simulink model "experiment_simulation"  (R2023b)
settings: Solver=VariableStepAuto  StartTime=0.0  StopTime=27  RelTol=1e-3
InitFcn:
  | parameters
model workspace (MAT data in the model file):
  trajectory_a = [-1.52409846931  1.70613035573  0.374243089925  1.5344612197  -0.302096275649  0.429029543536  -1.71694567009  1.69908972473  0.568317664567  -1.58200132841; 0.800900294758  -0.416782684687  -1.66038099689  -1.1420845298  -1.00480440985  -1.09338745015  0.812017564072  1.01661034087  0.189146535455  0.213933679737; 0.522291166812  1.94182780206  0.53711281193  0.401822450123  1.63674782832  0.283346535529  -0.658320315012  1.82855663324  -0.240307510879  0.406170374063; 0.881049446282  0.715113366686  -1.14896395959  -1.67350649982  -0.902082368458  1.47007354587  0.23742826959  -0.141488915891  -0.278796396878  1.09594368008; 0.615681685123  0.630917086666  -1.35591638166  -0.270492692225  0.0203443374221  -0.49867087628  -0.0785110876565  -0.630314388932  1.10858576056  -0.464224550441; 0.846225707965  -0.0762663704322  0.916720888486  1.75023695585  0.0690176102037  1.61227499451  -1.12722943148  1.49287736069  -1.66922827228  -0.138386333717; -1.91228070877  1.23312220014  -1.28316199684  -1.33843101258  -1.27358613135  0.765746253245  -1.14494592309  -0.807580560907  1.07334058824  0.00460037858408]
  trajectory_b = [1.63785922603  -1.76858838765  -0.252992287028  0.289018982285  0.260268639109  1.29526626891  -1.49560469007  -0.799532889865  -1.99151190067  1.80442943156; 1.06519745333  1.00521664875  -1.44454065144  -0.602721829429  -1.39463775801  -0.0131172869683  1.23460901165  0.531475173765  0.753605990771  0.558280871421; 0.917286904974  1.43938283234  0.507821517658  -1.27763450836  0.29322618533  -1.34573537446  1.6242069423  -1.69062885947  -0.645861399433  0.322470189589; -0.0990593700309  1.2212819449  0.123112563899  -1.09075867343  0.837939900786  -1.40546978718  0.632464724894  0.53593019156  -1.08277499414  -1.27108793891; -1.33458996905  -1.40157163353  -1.18901040903  1.81983560726  -1.93636664476  1.83005740068  -1.89723085852  1.88444265238  -0.809617292966  0.100292316878; 1.44935684592  1.58561961386  -1.24395777836  0.642878229792  1.76492375149  1.90282850268  -1.56825898793  -1.28440308791  0.986205708528  -1.80212590987; -1.71486047215  -0.0434979217147  1.39957528496  1.98816577551  -1.98242954967  0.170429856236  1.44539270567  1.63655609788  1.38140224911  1.51549153855]
values from neighbouring files (symbols this model uses):
  m = length(U)-1    [bspline_findspan.m]
  param_robot = load_mu(param_robot, mu)    [parameters.m]
undefined symbols (not defined in the file or in its folder): par, param_initial_condition, param_sensor, X, Y, Z
libraries: nesl_utility x308, sm_lib x269, simulink_extras x1
(part 1 of 4)
settings Model: Creator=cha  LastModifiedBy=simon
settings SolverCC: AlgebraicLoopSolver=TrustRegion
settings DataIOCC: ReturnWorkspaceOutputs=off
settings DebuggingCC: UnconnectedLineMsg=warning  ArithmeticOperatorsInVariantConditions=warning
settings ModelReferenceCC: EnableRefExpFcnMdlSchedulingChecks=on
settings SFSimCC: SimUseLocalCustomCode=off  CustomCodeUndefinedFunction=UseInterfaceOnly
settings RTWCC: RTWUseLocalCustomCode=off
settings ExplorerConfigSet: InternalSimMechanicsExplorerSettings="<ExplorerConfiguration><canonicalview>default</canonicalview><AnimationSetting><BasePlaybackSpeed>1.0</BasePlaybackSpeed><PlaybackSpeedFactor>1.0</PlaybackSpeedFactor></AnimationSetting><TilePanel><TileInfo><Tiles Columns=\"1\" Count=\"1\" Rows=\"1\"><Column Weight=\"1\"/><Row Weight=\"1\"/><Tile Height=\"1\" Width=\"1\" X=\"0\" Y=\"0\"/></Tiles></TileInfo><SceneInfo><SceneViewer><BGColor><R>0.60000002384185791</R><G>0.60000002384185791</G><B>0.60000002384185791</B></BGColor><Camera><DoPerspective>off</DoPerspective><Position><X>0.880405044047670393</X><Y>-0.700942246579231321</Y><Z>1.1419415318535151</Z></Position><Center><X>0.329533173940033675</X><Y>0.0559357238790175043</Y><Z>0.725925616444012989</Z></Center><Up><X>-0.2202813222044534</X><Y>0.341822804085735843</Y><Z>0.913582678083830313</Z></Up><ViewLimDist>1</ViewLimDist><YLim>0.787222366901565107</YLim><XLim>1.5531684536166015</XLim></Camera></SceneViewer></SceneInfo></TilePanel><MechEditorPanel><Cameras/><GfxPanelCameraMap/><VideoCreator><PlaybackSpeedRatio>1.0</PlaybackSpeedRatio><FrameRate>30</FrameRate><VideoFormat>Motion JPEG AVI</VideoFormat><FrameSize>auto</FrameSize></VideoCreator></MechEditorPanel></ExplorerConfiguration>"

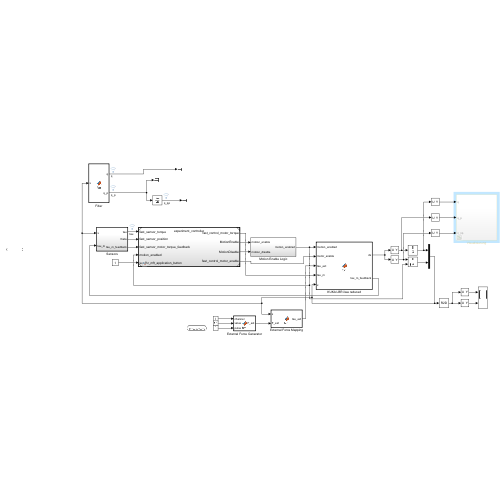
[thumbnail: Simulink's stored preview of the top-level diagram]
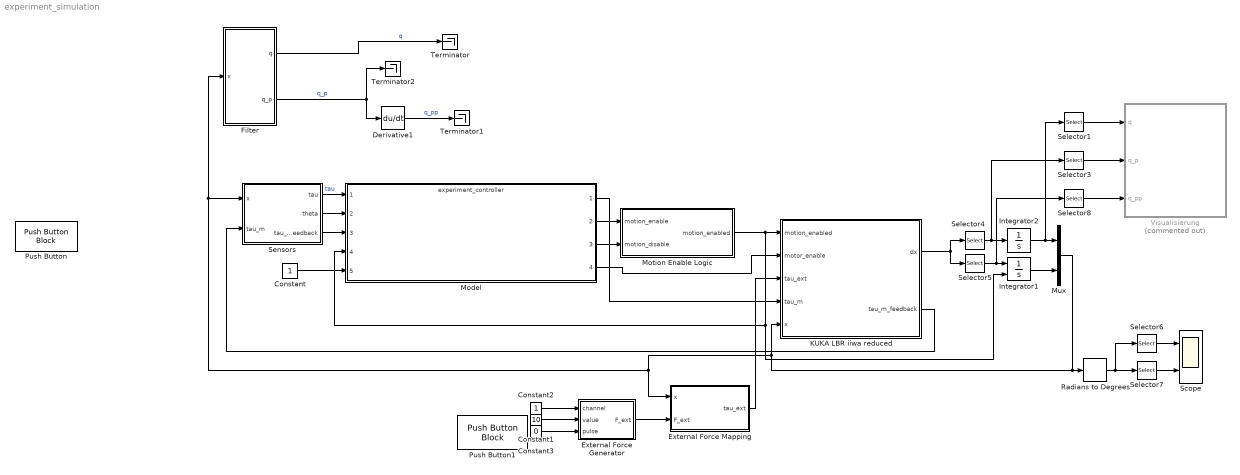
== system experiment_simulation ==
  Constant : Constant
  Constant1 : Constant  Value=10
  Constant2 : Constant
  Constant3 : Constant  Value=0
  Derivative1 : Derivative
  External Force Generator : MATLAB Function  TreatAsAtomicUnit=on
  External Force Mapping : MATLAB Function  TreatAsAtomicUnit=on
  Filter : MATLAB Function  TreatAsAtomicUnit=on
  Integrator1 : Integrator  ExternalReset=falling  InitialCondition=[param_initial_condition.q__p_0;param_initial_condition.theta__p_0]
  Integrator2 : Integrator  InitialCondition=[param_initial_condition.q__0;param_initial_condition.theta__0]
  KUKA LBR iiwa reduced : MATLAB Function  TreatAsAtomicUnit=on
  Model : ModelReference  ModelNameDialog=experiment_controller.slx  SimulationMode=Normal  ModelReferenceVersion=11.12
  Motion Enable Logic : Subsystem
  Mux : Mux  Inputs=2
  Push Button : PushButtonBlock  ButtonText=MFT Button  OffValue=1.000000
  Push Button1 : PushButtonBlock  ButtonText=Force/Torque
  Radians to Degrees : simulink_extras/Transformations/Radians to Degrees
  Scope : Scope  NumInputPorts=2
  Selector1 : Selector  InputPortWidth=14  IndexOptions=Index vector (dialog)  Indices=[1:7]  OutputSizes=1
  Selector3 : Selector  InputPortWidth=14  IndexOptions=Index vector (dialog)  Indices=[1:7]  OutputSizes=1
  Selector4 : Selector  InputPortWidth=28  IndexOptions=Index vector (dialog)  Indices=[1:14]  OutputSizes=1
  Selector5 : Selector  InputPortWidth=28  IndexOptions=Index vector (dialog)  Indices=[15:28]  OutputSizes=1
  Selector6 : Selector  InputPortWidth=28  IndexOptions=Index vector (dialog)  Indices=[1:7]  OutputSizes=1
  Selector7 : Selector  InputPortWidth=28  IndexOptions=Index vector (dialog)  Indices=[15:21]  OutputSizes=1
  Selector8 : Selector  InputPortWidth=14  IndexOptions=Index vector (dialog)  Indices=[1:7]  OutputSizes=1
  Sensors : Subsystem  TreatAsAtomicUnit=on  SystemSampleTime=param_sensor.T_a
  Terminator : Terminator
  Terminator1 : Terminator
  Terminator2 : Terminator
  Visualisierung : Subsystem  Commented=on
  wires:
  Sensors/1(tau) -> Model/1  "tau"
  Model/1 -> KUKA LBR iiwa reduced/4(tau_m)
  Mux/1 -> Radians to Degrees/1, Filter/1(x), Sensors/1(x), External Force Mapping/1(x), KUKA LBR iiwa reduced/5(x)
  Sensors/2(theta) -> Model/2
  KUKA LBR iiwa reduced/1(dx) -> Selector4/1, Selector5/1
  Sensors/3(tau_m_feedback) -> Model/3
  External Force Mapping/1(tau_ext) -> KUKA LBR iiwa reduced/3(tau_ext)
  Model/4 -> KUKA LBR iiwa reduced/2(motor_enable)
  Integrator2/1 -> Selector1/1, Mux/1
  Integrator1/1 -> Mux/2
  Selector5/1 -> Selector8/1, Integrator1/1
  Motion Enable Logic/1(motion_enabled) -> Integrator1/2, Model/4, KUKA LBR iiwa reduced/1(motion_enabled)
  Model/2 -> Motion Enable Logic/1(motion_enable)
  Model/3 -> Motion Enable Logic/2(motion_disable)
  KUKA LBR iiwa reduced/2(tau_m_feedback) -> Sensors/2(tau_m)
  Selector7/1 -> Scope/2
  Selector6/1 -> Scope/1
  External Force Generator/1(F_ext) -> External Force Mapping/2(F_ext)
  Constant1/1 -> External Force Generator/2(value)
  Constant2/1 -> External Force Generator/1(channel)
  Constant3/1 -> External Force Generator/3(pulse)
  Radians to Degrees/1 -> Selector7/1, Selector6/1
  Constant/1 -> Model/5
  Selector4/1 -> Selector3/1, Integrator2/1
  Selector1/1 -> Visualisierung/1(q)
  Selector3/1 -> Visualisierung/2(q_p)
  Selector8/1 -> Visualisierung/3(q_pp)
  Filter/2(q_p) -> Derivative1/1, Terminator2/1  "q_p"
  Filter/1(q) -> Terminator/1  "q"
  Derivative1/1 -> Terminator1/1  "q_pp"

== system experiment_simulation/Motion Enable Logic ==
  motion_enable : Inport
  motion_disable : Inport  Port=2
  Memory : Memory
  Motion Enable Logic : MATLAB Function  TreatAsAtomicUnit=on
  motion_enabled : Outport  VectorParamsAs1DForOutWhenUnconnected=off
  wires:
  motion_disable/1 -> Motion Enable Logic/2(motion_disable)
  motion_enable/1 -> Motion Enable Logic/1(motion_enable)
  Motion Enable Logic/1(motion_enabled) -> Memory/1
  Memory/1 -> motion_enabled/1

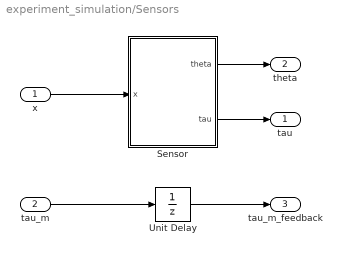
== system experiment_simulation/Sensors ==
  x : Inport
  tau_m : Inport  Port=2
  Sensor : MATLAB Function  SystemSampleTime=param_sensor.T_a
  Unit Delay : UnitDelay  SampleTime=-1  HasFrameUpgradeWarning=on
  tau : Outport  VectorParamsAs1DForOutWhenUnconnected=off
  theta : Outport  Port=2  VectorParamsAs1DForOutWhenUnconnected=off
  tau_m_feedback : Outport  Port=3  VectorParamsAs1DForOutWhenUnconnected=off
  wires:
  Sensor/1(theta) -> theta/1
  Sensor/2(tau) -> tau/1
  x/1 -> Sensor/1(x)
  tau_m/1 -> Unit Delay/1
  Unit Delay/1 -> tau_m_feedback/1

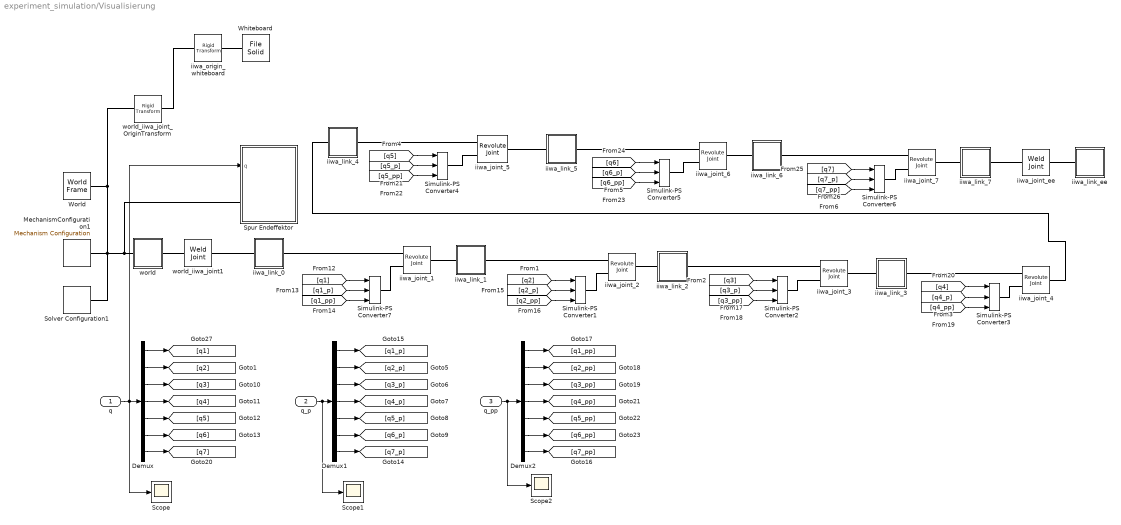
== system experiment_simulation/Visualisierung ==
  q : Inport
  q_p : Inport  Port=2
  q_pp : Inport  Port=3
  Demux : Demux  Outputs=7
  Demux1 : Demux  Outputs=7
  Demux2 : Demux  Outputs=7
  MechanismConfiguration1 : sm_lib/Utilities/Mechanism Configuration  UniformGravity=Constant  GravityVector=param_robot.g_vis  GravityVectorUnits=m/s^2  LinearizationDelta=0.001  JointModeTransitionNonlinearIterations=2
  Scope : Scope
  Scope1 : Scope
  Scope2 : Scope
  Simulink-PS Converter{1..7} (7 alike) : nesl_utility/Simulink-PS Converter  PhysicalDomain=network_engine_domain  SubClassName=ps_input  LeftPortType=input  RightPortType=output  PseudoPeriodic=off  Frequencies=[]  NoiseDistribution=none  NoiseParameters=[]  Unit=1  AffineConversion=off  FilteringAndDerivatives=provide  SimscapeFilterOrder=2  InputFilterTimeConstant=0.001  UdotUserProvided=2
  Solver Configuration1 : nesl_utility/Solver Configuration  PhysicalDomain=network_engine_domain  SubClassName=solver  LeftPortType=input  RightPortType=generic  Tones=[]  Harmonics=[]  SimulateNoise=off  Profile=off  UseLocalSampling=off  EnableSwitchedLinearOptims=on  FrequencyDomain=off  UseCCode=off  RelTol=0.001  AbsTol=1e-06  MinStep=1e-09  ToWorkspace=off  RevertToSquareIcSolve=off  NumHomotopyIterations=100  PhasorMode=off  PhasorModeNumHarmonics=1  ConsistencySolver=NEWTON_FTOL  IndexReductionMethod=DerivativeReplacement  DoDC=off  ResidualTolerance=1e-09  ConsistencyTolSource=GLOBAL  ConsistencyAbsTol=0.001  ConsistencyRelTol=0.001  ConsistencyTolFactor=0.001  UseLocalSolver=off  LocalSolverChoice=NE_BACKWARD_EULER_ADVANCER  ResolveIndetEquations=on  FunctionEvalNumThread=1  LocalSolverSampleTime=0.001  DoFixedCost=off  MaxNonlinIter=3  MaxModeIter=2  ComputeImpulses=off  ImpulseIterations=2  LinearAlgebra=Sparse  LinearAlgebraNumThread=0  EquationFormulation=NE_TIME_EF  DelaysMemoryBudget=1024  AutomaticFiltering=on  FilteringTimeConstant=0.001  PartitionStorageMethod=AS_NEEDED  PartitionMemoryBudget=1024  PartitionMethod=FAST  MultibodyUseLocalSolver=off  MultibodyLocalSolverChoice=ODE1  MultibodyLocalSolverSampleTime=0.001
  Spur Endeffektor : Subsystem
  Whiteboard : sm_lib/Body Elements/File Solid  ExtGeomFileName=.\kukalbriiwa_model\meshes\Whiteboard.stl  UnitType=Custom  ExtGeomFileUnits=mm  StepReaderType=HEX  ExportConvexHullGeometry=off  InertiaType=Custom  Mass=0  MassUnits=kg  CenterOfMass=[0, 0, 0]  CenterOfMassUnits=m  MomentsOfInertia=[0, 0, 0]  MomentsOfInertiaUnits=kg*m^2  ProductsOfInertia=[0, 0, 0]  ProductsOfInertiaUnits=kg*m^2  BasedOnType=Density  Density=1000  DensityUnits=kg/m^3  DoExposeReferenceFrame=on  SerializedFrames=<Frames/>  GraphicType=FromGeometry  MarkerShape=Sphere  MarkerSize=10  GraphicVisPropType=SimpleVisualProperties  GraphicDiffuseColor=par.Wb_col  GraphicSpecularColor=[0.5 0.5 0.5 1.0]  GraphicAmbientColor=[0.15 0.15 0.15 1.0]  GraphicEmissiveColor=[0.0 0.0 0.0 1.0]  GraphicShininess=75  GraphicOpacity=par.Wb_opa
  World : sm_lib/Frames and Transforms/World Frame
  iiwa_joint_{1..7} (7 alike) : sm_lib/Joints/Revolute Joint  JointMode=Normal  SenseConstraintForce=off  SenseConstraintForceX=off  SenseConstraintForceY=off  SenseConstraintForceZ=off  SenseConstraintTorque=off  SenseConstraintTorqueX=off  SenseConstraintTorqueY=off  SenseConstraintTorqueZ=off  SenseTotalForce=off  SenseTotalForceX=off  SenseTotalForceY=off  SenseTotalForceZ=off  SenseTotalTorque=off  SenseTotalTorqueX=off  SenseTotalTorqueY=off  SenseTotalTorqueZ=off  CompositeWrenchDir=FollowerOnBase  CompositeWrenchFrame=BaseFrame  EquilibriumPosition=0  EquilibriumPositionUnits=deg  SpringStiffness=0  SpringStiffnessUnits=N*m/deg  DampingCoefficient=0  DampingCoefficientUnits=m^2*kg/s/rad  TorqueActuationMode=ComputedTorque  MotionActuationMode=InputMotion  SensePosition=off  SenseVelocity=off  SenseAcceleration=off  SenseTorqueForce=off  SenseLowerLimitTorqueForce=off  SenseUpperLimitTorqueForce=off  LowerLimitSpecify=off  LowerLimitBound=-90  LowerLimitBoundUnits=deg  LowerLimitStiffness=1e4  LowerLimitStiffnessUnits=N*m/deg  LowerLimitDamping=10  LowerLimitDampingUnits=N*m/(deg/s)  LowerLimitTransitionRegionWidth=0.1  LowerLimitTransitionRegionWidthUnits=deg  UpperLimitSpecify=off  UpperLimitBound=90  UpperLimitBoundUnits=deg  UpperLimitStiffness=1e4  UpperLimitStiffnessUnits=N*m/deg  UpperLimitDamping=10  UpperLimitDampingUnits=N*m/(deg/s)  UpperLimitTransitionRegionWidth=0.1  UpperLimitTransitionRegionWidthUnits=deg  PositionTargetSpecify=on  PositionTargetPriority=High  PositionTargetValue=0  PositionTargetValueUnits=rad  VelocityTargetSpecify=off  VelocityTargetPriority=High  VelocityTargetValue=0  VelocityTargetValueUnits=deg/s
  iiwa_joint_ee : sm_lib/Joints/Weld Joint  JointMode=Normal  SenseConstraintForce=off  SenseConstraintForceX=off  SenseConstraintForceY=off  SenseConstraintForceZ=off  SenseConstraintTorque=off  SenseConstraintTorqueX=off  SenseConstraintTorqueY=off  SenseConstraintTorqueZ=off  SenseTotalForce=off  SenseTotalForceX=off  SenseTotalForceY=off  SenseTotalForceZ=off  SenseTotalTorque=off  SenseTotalTorqueX=off  SenseTotalTorqueY=off  SenseTotalTorqueZ=off  CompositeWrenchDir=FollowerOnBase  CompositeWrenchFrame=BaseFrame
  iiwa_link_0 : Subsystem
  iiwa_link_1 : Subsystem
  iiwa_link_2 : Subsystem
  iiwa_link_3 : Subsystem
  iiwa_link_4 : Subsystem
  iiwa_link_5 : Subsystem
  iiwa_link_6 : Subsystem
  iiwa_link_7 : Subsystem
  iiwa_link_ee : Subsystem
  iiwa_origin_whiteboard : sm_lib/Frames and Transforms/Rigid Transform  TranslationMethod=Cartesian  TranslationStandardOffset=0  TranslationStandardOffsetUnits=m  TranslationStandardAxis=+Z  TranslationCartesianOffset=par.T_0w(1:3,4)  TranslationCartesianOffsetUnits=m  TranslationROffset=0  TranslationROffsetUnits=m  TranslationZOffset=0  TranslationZOffsetUnits=m  TranslationThetaOffset=0  TranslationThetaOffsetUnits=deg  RotationMethod=RotationMatrix  RotationAngleUnits=deg  RotationStandardAxis=+Z  RotationAngle=0.0  RotationArbitraryAxis=[0 0 1]  FollAlignAxisA=+X  BaseAlignAxisA=+Y  FollAlignAxisB=+Y  BaseAlignAxisB=+Z  RotationSequenceAxes=BaseAxes  RotationSequence=XYZ  RotationSequenceAngles=[0, 0, 0]  RotationSequenceAnglesUnits=rad  RotationMatrix=par.R_0w  Quaternion=[1 0 0 0]
  world : Subsystem
  world_iiwa_joint1 : sm_lib/Joints/Weld Joint  JointMode=Normal  SenseConstraintForce=off  SenseConstraintForceX=off  SenseConstraintForceY=off  SenseConstraintForceZ=off  SenseConstraintTorque=off  SenseConstraintTorqueX=off  SenseConstraintTorqueY=off  SenseConstraintTorqueZ=off  SenseTotalForce=off  SenseTotalForceX=off  SenseTotalForceY=off  SenseTotalForceZ=off  SenseTotalTorque=off  SenseTotalTorqueX=off  SenseTotalTorqueY=off  SenseTotalTorqueZ=off  CompositeWrenchDir=FollowerOnBase  CompositeWrenchFrame=BaseFrame
  world_iiwa_joint_OriginTransform : sm_lib/Frames and Transforms/Rigid Transform  TranslationMethod=Cartesian  TranslationStandardOffset=0  TranslationStandardOffsetUnits=m  TranslationStandardAxis=+Z  TranslationCartesianOffset=param_robot.p_0  TranslationCartesianOffsetUnits=m  TranslationROffset=0  TranslationROffsetUnits=m  TranslationZOffset=0  TranslationZOffsetUnits=m  TranslationThetaOffset=0  TranslationThetaOffsetUnits=deg  RotationMethod=RotationMatrix  RotationAngleUnits=deg  RotationStandardAxis=+Z  RotationAngle=0.0  RotationArbitraryAxis=[0 0 1]  FollAlignAxisA=+X  BaseAlignAxisA=+Y  FollAlignAxisB=+Y  BaseAlignAxisB=+Z  RotationSequenceAxes=BaseAxes  RotationSequence=XYZ  RotationSequenceAngles=[0, 0, 0]  RotationSequenceAnglesUnits=rad  RotationMatrix=param_robot.R_0  Quaternion=[1 0 0 0]
  wires:
  Demux/7 -> [q7]
  Demux/6 -> [q6]
  Demux/5 -> [q5]
  Demux/4 -> [q4]
  Demux/3 -> [q3]
  Demux/2 -> [q2]
  Demux/1 -> [q1]
  q_p/1 -> Scope1/1, Demux1/1
  Demux1/1 -> [q1_p]
  Demux1/2 -> [q2_p]
  Demux1/3 -> [q3_p]
  Demux1/4 -> [q4_p]
  Demux1/5 -> [q5_p]
  Demux1/6 -> [q6_p]
  Demux1/7 -> [q7_p]
  Demux2/7 -> [q7_pp]
  Demux2/6 -> [q6_pp]
  Demux2/5 -> [q5_pp]
  Demux2/4 -> [q4_pp]
  Demux2/3 -> [q3_pp]
  Demux2/2 -> [q2_pp]
  Demux2/1 -> [q1_pp]
  q_pp/1 -> Scope2/1, Demux2/1
  [q2] -> Simulink-PS Converter1/1
  [q7_p] -> Simulink-PS Converter6/2
  q/1 -> Spur Endeffektor/1(q), Scope/1, Demux/1
  [q4_pp] -> Simulink-PS Converter3/3
  [q3_p] -> Simulink-PS Converter2/2
  [q5_p] -> Simulink-PS Converter4/2
  [q5_pp] -> Simulink-PS Converter4/3
  [q2_pp] -> Simulink-PS Converter1/3
  [q6_p] -> Simulink-PS Converter5/2
  [q6_pp] -> Simulink-PS Converter5/3
  [q1] -> Simulink-PS Converter7/1
  [q4_p] -> Simulink-PS Converter3/2
  [q7] -> Simulink-PS Converter6/1
  [q3] -> Simulink-PS Converter2/1
  [q2_p] -> Simulink-PS Converter1/2
  [q6] -> Simulink-PS Converter5/1
  [q4] -> Simulink-PS Converter3/1
  [q1_pp] -> Simulink-PS Converter7/3
  [q5] -> Simulink-PS Converter4/1
  [q1_p] -> Simulink-PS Converter7/2
  [q7_pp] -> Simulink-PS Converter6/3
  [q3_pp] -> Simulink-PS Converter2/3
  connections:
  world/LConn1 -- Spur Endeffektor/LConn1 -- Solver Configuration1/RConn1 -- MechanismConfiguration1/RConn1 -- world_iiwa_joint_OriginTransform/LConn1 -- World/RConn1
  iiwa_origin_whiteboard/LConn1 -- world_iiwa_joint_OriginTransform/RConn1
  iiwa_origin_whiteboard/RConn1 -- Whiteboard/RConn1
  iiwa_link_0/LConn1 -- world_iiwa_joint1/RConn1
  iiwa_joint_3/LConn2 -- Simulink-PS Converter2/RConn1
  world/RConn1 -- world_iiwa_joint1/LConn1
  iiwa_joint_3/RConn1 -- iiwa_link_3/LConn1
  Simulink-PS Converter5/RConn1 -- iiwa_joint_6/LConn2
  iiwa_joint_2/RConn1 -- iiwa_link_2/LConn1
  iiwa_link_0/RConn1 -- iiwa_joint_1/LConn1
  Simulink-PS Converter4/RConn1 -- iiwa_joint_5/LConn2
  iiwa_joint_6/LConn1 -- iiwa_link_5/RConn1
  iiwa_joint_7/RConn1 -- iiwa_link_7/LConn1
  iiwa_joint_1/LConn2 -- Simulink-PS Converter7/RConn1
  iiwa_joint_6/RConn1 -- iiwa_link_6/LConn1
  Simulink-PS Converter6/RConn1 -- iiwa_joint_7/LConn2
  iiwa_joint_4/RConn1 -- iiwa_link_4/LConn1
  iiwa_joint_5/RConn1 -- iiwa_link_5/LConn1
  iiwa_joint_5/LConn1 -- iiwa_link_4/RConn1
  iiwa_joint_1/RConn1 -- iiwa_link_1/LConn1
  iiwa_joint_7/LConn1 -- iiwa_link_6/RConn1
  Simulink-PS Converter1/RConn1 -- iiwa_joint_2/LConn2
  iiwa_joint_ee/LConn1 -- iiwa_link_7/RConn1
  iiwa_joint_4/LConn1 -- iiwa_link_3/RConn1
  iiwa_joint_3/LConn1 -- iiwa_link_2/RConn1
  Simulink-PS Converter3/RConn1 -- iiwa_joint_4/LConn2
  iiwa_joint_2/LConn1 -- iiwa_link_1/RConn1
  iiwa_joint_ee/RConn1 -- iiwa_link_ee/LConn1

== system experiment_simulation/Visualisierung/Spur Endeffektor ==
  q : Inport
  MATLAB Function : MATLAB Function  TreatAsAtomicUnit=on
  Visualisierung Punkte : Subsystem
  delta : Constant  Value=par.vis_point.delta
  start : Constant
  Conn1 : PMIOPort  Side=Left
  wires:
  MATLAB Function/1(p1) -> Visualisierung Punkte/1(p1)
  MATLAB Function/2(p2) -> Visualisierung Punkte/2(p2)
  MATLAB Function/3(p3) -> Visualisierung Punkte/3(p3)
  MATLAB Function/4(p4) -> Visualisierung Punkte/4(p4)
  MATLAB Function/5(p5) -> Visualisierung Punkte/5(p5)
  MATLAB Function/6(p6) -> Visualisierung Punkte/6(p6)
  MATLAB Function/7(p7) -> Visualisierung Punkte/7(p7)
  MATLAB Function/8(p8) -> Visualisierung Punkte/8(p8)
  MATLAB Function/9(p9) -> Visualisierung Punkte/9(p9)
  MATLAB Function/10(p10) -> Visualisierung Punkte/10(p10)
  MATLAB Function/11(p11) -> Visualisierung Punkte/11(p11)
  MATLAB Function/12(p12) -> Visualisierung Punkte/12(p12)
  MATLAB Function/13(p13) -> Visualisierung Punkte/13(p13)
  MATLAB Function/14(p14) -> Visualisierung Punkte/14(p14)
  MATLAB Function/15(p15) -> Visualisierung Punkte/15(p15)
  MATLAB Function/16(p16) -> Visualisierung Punkte/16(p16)
  MATLAB Function/17(p17) -> Visualisierung Punkte/17(p17)
  MATLAB Function/18(p18) -> Visualisierung Punkte/18(p18)
  MATLAB Function/19(p19) -> Visualisierung Punkte/19(p19)
  MATLAB Function/20(p20) -> Visualisierung Punkte/20(p20)
  MATLAB Function/21(p21) -> Visualisierung Punkte/21(p21)
  MATLAB Function/22(p22) -> Visualisierung Punkte/22(p22)
  MATLAB Function/23(p23) -> Visualisierung Punkte/23(p23)
  MATLAB Function/24(p24) -> Visualisierung Punkte/24(p24)
  MATLAB Function/25(p25) -> Visualisierung Punkte/25(p25)
  MATLAB Function/26(p26) -> Visualisierung Punkte/26(p26)
  MATLAB Function/27(p27) -> Visualisierung Punkte/27(p27)
  MATLAB Function/28(p28) -> Visualisierung Punkte/28(p28)
  MATLAB Function/29(p29) -> Visualisierung Punkte/29(p29)
  MATLAB Function/30(p30) -> Visualisierung Punkte/30(p30)
  MATLAB Function/31(p31) -> Visualisierung Punkte/31(p31)
  MATLAB Function/32(p32) -> Visualisierung Punkte/32(p32)
  MATLAB Function/33(p33) -> Visualisierung Punkte/33(p33)
  MATLAB Function/34(p34) -> Visualisierung Punkte/34(p34)
  MATLAB Function/35(p35) -> Visualisierung Punkte/35(p35)
  MATLAB Function/36(p36) -> Visualisierung Punkte/36(p36)
  MATLAB Function/37(p37) -> Visualisierung Punkte/37(p37)
  MATLAB Function/38(p38) -> Visualisierung Punkte/38(p38)
  MATLAB Function/39(p39) -> Visualisierung Punkte/39(p39)
  MATLAB Function/40(p40) -> Visualisierung Punkte/40(p40)
  MATLAB Function/41(p41) -> Visualisierung Punkte/41(p41)
  MATLAB Function/42(p42) -> Visualisierung Punkte/42(p42)
  MATLAB Function/43(p43) -> Visualisierung Punkte/43(p43)
  MATLAB Function/44(p44) -> Visualisierung Punkte/44(p44)
  MATLAB Function/45(p45) -> Visualisierung Punkte/45(p45)
  MATLAB Function/46(p46) -> Visualisierung Punkte/46(p46)
  MATLAB Function/47(p47) -> Visualisierung Punkte/47(p47)
  MATLAB Function/48(p48) -> Visualisierung Punkte/48(p48)
  MATLAB Function/49(p49) -> Visualisierung Punkte/49(p49)
  MATLAB Function/50(p50) -> Visualisierung Punkte/50(p50)
  MATLAB Function/51(p51) -> Visualisierung Punkte/51(p51)
  MATLAB Function/52(p52) -> Visualisierung Punkte/52(p52)
  MATLAB Function/53(p53) -> Visualisierung Punkte/53(p53)
  MATLAB Function/54(p54) -> Visualisierung Punkte/54(p54)
  MATLAB Function/55(p55) -> Visualisierung Punkte/55(p55)
  MATLAB Function/56(p56) -> Visualisierung Punkte/56(p56)
  MATLAB Function/57(p57) -> Visualisierung Punkte/57(p57)
  MATLAB Function/58(p58) -> Visualisierung Punkte/58(p58)
  MATLAB Function/59(p59) -> Visualisierung Punkte/59(p59)
  MATLAB Function/60(p60) -> Visualisierung Punkte/60(p60)
  MATLAB Function/61(p61) -> Visualisierung Punkte/61(p61)
  MATLAB Function/62(p62) -> Visualisierung Punkte/62(p62)
  MATLAB Function/63(p63) -> Visualisierung Punkte/63(p63)
  MATLAB Function/64(p64) -> Visualisierung Punkte/64(p64)
  MATLAB Function/65(p65) -> Visualisierung Punkte/65(p65)
  MATLAB Function/66(p66) -> Visualisierung Punkte/66(p66)
  MATLAB Function/67(p67) -> Visualisierung Punkte/67(p67)
  MATLAB Function/68(p68) -> Visualisierung Punkte/68(p68)
  MATLAB Function/69(p69) -> Visualisierung Punkte/69(p69)
  MATLAB Function/70(p70) -> Visualisierung Punkte/70(p70)
  MATLAB Function/71(p71) -> Visualisierung Punkte/71(p71)
  MATLAB Function/72(p72) -> Visualisierung Punkte/72(p72)
  MATLAB Function/73(p73) -> Visualisierung Punkte/73(p73)
  MATLAB Function/74(p74) -> Visualisierung Punkte/74(p74)
  MATLAB Function/75(p75) -> Visualisierung Punkte/75(p75)
  MATLAB Function/76(p76) -> Visualisierung Punkte/76(p76)
  MATLAB Function/77(p77) -> Visualisierung Punkte/77(p77)
  MATLAB Function/78(p78) -> Visualisierung Punkte/78(p78)
  MATLAB Function/79(p79) -> Visualisierung Punkte/79(p79)
  MATLAB Function/80(p80) -> Visualisierung Punkte/80(p80)
  MATLAB Function/81(p81) -> Visualisierung Punkte/81(p81)
  MATLAB Function/82(p82) -> Visualisierung Punkte/82(p82)
  MATLAB Function/83(p83) -> Visualisierung Punkte/83(p83)
  MATLAB Function/84(p84) -> Visualisierung Punkte/84(p84)
  MATLAB Function/85(p85) -> Visualisierung Punkte/85(p85)
  MATLAB Function/86(p86) -> Visualisierung Punkte/86(p86)
  MATLAB Function/87(p87) -> Visualisierung Punkte/87(p87)
  MATLAB Function/88(p88) -> Visualisierung Punkte/88(p88)
  MATLAB Function/89(p89) -> Visualisierung Punkte/89(p89)
  MATLAB Function/90(p90) -> Visualisierung Punkte/90(p90)
  MATLAB Function/91(p91) -> Visualisierung Punkte/91(p91)
  MATLAB Function/92(p92) -> Visualisierung Punkte/92(p92)
  MATLAB Function/93(p93) -> Visualisierung Punkte/93(p93)
  MATLAB Function/94(p94) -> Visualisierung Punkte/94(p94)
  MATLAB Function/95(p95) -> Visualisierung Punkte/95(p95)
  MATLAB Function/96(p96) -> Visualisierung Punkte/96(p96)
  MATLAB Function/97(p97) -> Visualisierung Punkte/97(p97)
  MATLAB Function/98(p98) -> Visualisierung Punkte/98(p98)
  MATLAB Function/99(p99) -> Visualisierung Punkte/99(p99)
  MATLAB Function/100(p100) -> Visualisierung Punkte/100(p100)
  delta/1 -> MATLAB Function/3(delta)
  q/1 -> MATLAB Function/1(q)
  start/1 -> MATLAB Function/2(start)
  connections:
  Conn1/RConn1 -- Visualisierung Punkte/LConn1

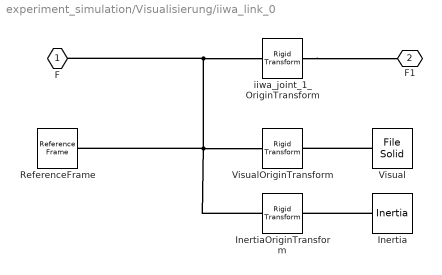
== system experiment_simulation/Visualisierung/iiwa_link_0 ==
  Inertia : sm_lib/Body Elements/Inertia  InertiaType=Custom  Mass=param_robot.link__0.m__0  MassUnits=kg  CenterOfMass=[0, 0, 0]  CenterOfMassUnits=m  MomentsOfInertia=param_robot.link__0.I__0  MomentsOfInertiaUnits=kg*m^2  ProductsOfInertia=[0, 0, 0]  ProductsOfInertiaUnits=kg*m^2  GraphicType=None  MarkerShape=Inertia  MarkerSize=20  GraphicVisPropType=SimpleVisualProperties  GraphicDiffuseColor=[0.5 0.5 0.5]  GraphicSpecularColor=[0.5 0.5 0.5 1.0]  GraphicAmbientColor=[0.15 0.15 0.15 1.0]  GraphicEmissiveColor=[0.0 0.0 0.0 1.0]  GraphicShininess=75  GraphicOpacity=1.0
  InertiaOriginTransform : sm_lib/Frames and Transforms/Rigid Transform  TranslationMethod=Cartesian  TranslationStandardOffset=0  TranslationStandardOffsetUnits=m  TranslationStandardAxis=+Z  TranslationCartesianOffset=param_robot.link__0.d__inertiaOrigin  TranslationCartesianOffsetUnits=m  TranslationROffset=0  TranslationROffsetUnits=m  TranslationZOffset=0  TranslationZOffsetUnits=m  TranslationThetaOffset=0  TranslationThetaOffsetUnits=deg  RotationMethod=RotationMatrix  RotationAngleUnits=deg  RotationStandardAxis=+Z  RotationAngle=0.0  RotationArbitraryAxis=[0 0 1]  FollAlignAxisA=+X  BaseAlignAxisA=+Y  FollAlignAxisB=+Y  BaseAlignAxisB=+Z  RotationSequenceAxes=BaseAxes  RotationSequence=XYZ  RotationSequenceAngles=[0, 0, 0]  RotationSequenceAnglesUnits=rad  RotationMatrix=param_robot.link__0.R__inertiaOrigin  Quaternion=[1 0 0 0]
  ReferenceFrame : sm_lib/Frames and Transforms/Reference Frame
  Visual : sm_lib/Body Elements/File Solid  ExtGeomFileName=.\kukalbriiwa_model\meshes\link_0.stl  UnitType=Custom  ExtGeomFileUnits=mm  StepReaderType=HEX  ExportConvexHullGeometry=off  InertiaType=Custom  Mass=0  MassUnits=kg  CenterOfMass=[0, 0, 0]  CenterOfMassUnits=m  MomentsOfInertia=[0, 0, 0]  MomentsOfInertiaUnits=kg*m^2  ProductsOfInertia=[0, 0, 0]  ProductsOfInertiaUnits=kg*m^2  BasedOnType=Density  Density=1000  DensityUnits=kg/m^3  DoExposeReferenceFrame=on  SerializedFrames=<Frames/>  GraphicType=FromGeometry  MarkerShape=Sphere  MarkerSize=10  GraphicVisPropType=SimpleVisualProperties  GraphicDiffuseColor=[0.4, 0.4, 0.4]  GraphicSpecularColor=[0.5 0.5 0.5 1.0]  GraphicAmbientColor=[0.15 0.15 0.15 1.0]  GraphicEmissiveColor=[0.0 0.0 0.0 1.0]  GraphicShininess=75  GraphicOpacity=1
  VisualOriginTransform : sm_lib/Frames and Transforms/Rigid Transform  TranslationMethod=Cartesian  TranslationStandardOffset=0  TranslationStandardOffsetUnits=m  TranslationStandardAxis=+Z  TranslationCartesianOffset=[0, 0, 0]  TranslationCartesianOffsetUnits=m  TranslationROffset=0  TranslationROffsetUnits=m  TranslationZOffset=0  TranslationZOffsetUnits=m  TranslationThetaOffset=0  TranslationThetaOffsetUnits=deg  RotationMethod=RotationSequence  RotationAngleUnits=deg  RotationStandardAxis=+Z  RotationAngle=0.0  RotationArbitraryAxis=[0 0 1]  FollAlignAxisA=+X  BaseAlignAxisA=+Y  FollAlignAxisB=+Y  BaseAlignAxisB=+Z  RotationSequenceAxes=BaseAxes  RotationSequence=XYZ  RotationSequenceAngles=[0, 0, 0]  RotationSequenceAnglesUnits=rad  RotationMatrix=[1 0 0; 0 1 0; 0 0 1]  Quaternion=[1 0 0 0]
  iiwa_joint_1_OriginTransform : sm_lib/Frames and Transforms/Rigid Transform  TranslationMethod=Cartesian  TranslationStandardOffset=0  TranslationStandardOffsetUnits=m  TranslationStandardAxis=+Z  TranslationCartesianOffset=param_robot.link__0.d__joint1  TranslationCartesianOffsetUnits=m  TranslationROffset=0  TranslationROffsetUnits=m  TranslationZOffset=0  TranslationZOffsetUnits=m  TranslationThetaOffset=0  TranslationThetaOffsetUnits=deg  RotationMethod=RotationMatrix  RotationAngleUnits=deg  RotationStandardAxis=+Z  RotationAngle=0.0  RotationArbitraryAxis=[0 0 1]  FollAlignAxisA=+X  BaseAlignAxisA=+Y  FollAlignAxisB=+Y  BaseAlignAxisB=+Z  RotationSequenceAxes=BaseAxes  RotationSequence=XYZ  RotationSequenceAngles=[0, 0, 0]  RotationSequenceAnglesUnits=rad  RotationMatrix=param_robot.link__0.R__joint1  Quaternion=[1 0 0 0]
  F : PMIOPort  Side=Left
  F1 : PMIOPort  Port=2  Side=Right
  connections:
  iiwa_joint_1_OriginTransform/RConn1 -- F1/RConn1
  Visual/RConn1 -- VisualOriginTransform/RConn1
  ReferenceFrame/RConn1 -- InertiaOriginTransform/LConn1 -- VisualOriginTransform/LConn1 -- F/RConn1 -- iiwa_joint_1_OriginTransform/LConn1
  Inertia/RConn1 -- InertiaOriginTransform/RConn1

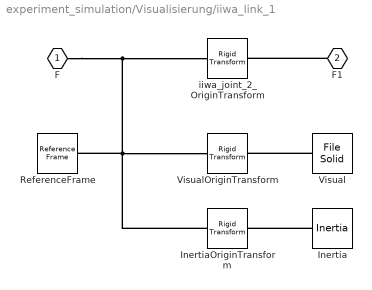
== system experiment_simulation/Visualisierung/iiwa_link_1 ==
  Inertia : sm_lib/Body Elements/Inertia  InertiaType=Custom  Mass=param_robot.link__1.m__1  MassUnits=kg  CenterOfMass=[0, 0, 0]  CenterOfMassUnits=m  MomentsOfInertia=param_robot.link__1.I__1  MomentsOfInertiaUnits=kg*m^2  ProductsOfInertia=[0, 0, 0]  ProductsOfInertiaUnits=kg*m^2  GraphicType=None  MarkerShape=Inertia  MarkerSize=20  GraphicVisPropType=SimpleVisualProperties  GraphicDiffuseColor=[0.5 0.5 0.5]  GraphicSpecularColor=[0.5 0.5 0.5 1.0]  GraphicAmbientColor=[0.15 0.15 0.15 1.0]  GraphicEmissiveColor=[0.0 0.0 0.0 1.0]  GraphicShininess=75  GraphicOpacity=1.0
  InertiaOriginTransform : sm_lib/Frames and Transforms/Rigid Transform  TranslationMethod=Cartesian  TranslationStandardOffset=0  TranslationStandardOffsetUnits=m  TranslationStandardAxis=+Z  TranslationCartesianOffset=param_robot.link__1.d__inertiaOrigin  TranslationCartesianOffsetUnits=m  TranslationROffset=0  TranslationROffsetUnits=m  TranslationZOffset=0  TranslationZOffsetUnits=m  TranslationThetaOffset=0  TranslationThetaOffsetUnits=deg  RotationMethod=RotationMatrix  RotationAngleUnits=deg  RotationStandardAxis=+Z  RotationAngle=0.0  RotationArbitraryAxis=[0 0 1]  FollAlignAxisA=+X  BaseAlignAxisA=+Y  FollAlignAxisB=+Y  BaseAlignAxisB=+Z  RotationSequenceAxes=BaseAxes  RotationSequence=XYZ  RotationSequenceAngles=[0, 0, 0]  RotationSequenceAnglesUnits=rad  RotationMatrix=param_robot.link__1.R__inertiaOrigin  Quaternion=[1 0 0 0]
  ReferenceFrame : sm_lib/Frames and Transforms/Reference Frame
  Visual : sm_lib/Body Elements/File Solid  ExtGeomFileName=.\kukalbriiwa_model\meshes\link_1.stl  UnitType=Custom  ExtGeomFileUnits=mm  StepReaderType=HEX  ExportConvexHullGeometry=off  InertiaType=Custom  Mass=0  MassUnits=kg  CenterOfMass=[0, 0, 0]  CenterOfMassUnits=m  MomentsOfInertia=[0, 0, 0]  MomentsOfInertiaUnits=kg*m^2  ProductsOfInertia=[0, 0, 0]  ProductsOfInertiaUnits=kg*m^2  BasedOnType=Density  Density=1000  DensityUnits=kg/m^3  DoExposeReferenceFrame=on  SerializedFrames=<Frames/>  GraphicType=FromGeometry  MarkerShape=Sphere  MarkerSize=10  GraphicVisPropType=SimpleVisualProperties  GraphicDiffuseColor=[1, 0.423529411765, 0.0392156862745]  GraphicSpecularColor=[0.5 0.5 0.5 1.0]  GraphicAmbientColor=[0.15 0.15 0.15 1.0]  GraphicEmissiveColor=[0.0 0.0 0.0 1.0]  GraphicShininess=75  GraphicOpacity=1
  VisualOriginTransform : sm_lib/Frames and Transforms/Rigid Transform  TranslationMethod=Cartesian  TranslationStandardOffset=0  TranslationStandardOffsetUnits=m  TranslationStandardAxis=+Z  TranslationCartesianOffset=[0, 0, 0]  TranslationCartesianOffsetUnits=m  TranslationROffset=0  TranslationROffsetUnits=m  TranslationZOffset=0  TranslationZOffsetUnits=m  TranslationThetaOffset=0  TranslationThetaOffsetUnits=deg  RotationMethod=RotationSequence  RotationAngleUnits=deg  RotationStandardAxis=+Z  RotationAngle=0.0  RotationArbitraryAxis=[0 0 1]  FollAlignAxisA=+X  BaseAlignAxisA=+Y  FollAlignAxisB=+Y  BaseAlignAxisB=+Z  RotationSequenceAxes=BaseAxes  RotationSequence=XYZ  RotationSequenceAngles=[0, 0, 0]  RotationSequenceAnglesUnits=rad  RotationMatrix=[1 0 0; 0 1 0; 0 0 1]  Quaternion=[1 0 0 0]
  iiwa_joint_2_OriginTransform : sm_lib/Frames and Transforms/Rigid Transform  TranslationMethod=Cartesian  TranslationStandardOffset=0  TranslationStandardOffsetUnits=m  TranslationStandardAxis=+Z  TranslationCartesianOffset=param_robot.link__1.d__joint2  TranslationCartesianOffsetUnits=m  TranslationROffset=0  TranslationROffsetUnits=m  TranslationZOffset=0  TranslationZOffsetUnits=m  TranslationThetaOffset=0  TranslationThetaOffsetUnits=deg  RotationMethod=RotationMatrix  RotationAngleUnits=deg  RotationStandardAxis=+Z  RotationAngle=0.0  RotationArbitraryAxis=[0 0 1]  FollAlignAxisA=+X  BaseAlignAxisA=+Y  FollAlignAxisB=+Y  BaseAlignAxisB=+Z  RotationSequenceAxes=BaseAxes  RotationSequence=XYZ  RotationSequenceAngles=[1.57079632679, 0, -3.141592653589587]  RotationSequenceAnglesUnits=rad  RotationMatrix=param_robot.link__1.R__joint2  Quaternion=[1 0 0 0]
  F : PMIOPort  Side=Left
  F1 : PMIOPort  Port=2  Side=Right
  connections:
  F1/RConn1 -- iiwa_joint_2_OriginTransform/RConn1
  Visual/RConn1 -- VisualOriginTransform/RConn1
  InertiaOriginTransform/LConn1 -- ReferenceFrame/RConn1 -- VisualOriginTransform/LConn1 -- F/RConn1 -- iiwa_joint_2_OriginTransform/LConn1
  Inertia/RConn1 -- InertiaOriginTransform/RConn1

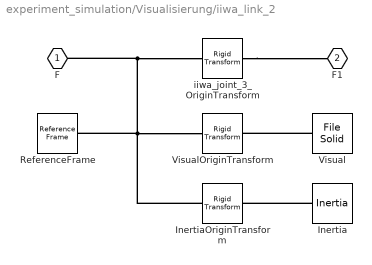
== system experiment_simulation/Visualisierung/iiwa_link_2 ==
  Inertia : sm_lib/Body Elements/Inertia  InertiaType=Custom  Mass=param_robot.link__2.m__2  MassUnits=kg  CenterOfMass=[0, 0, 0]  CenterOfMassUnits=m  MomentsOfInertia=param_robot.link__2.I__2  MomentsOfInertiaUnits=kg*m^2  ProductsOfInertia=[0, 0, 0]  ProductsOfInertiaUnits=kg*m^2  GraphicType=None  MarkerShape=Inertia  MarkerSize=20  GraphicVisPropType=SimpleVisualProperties  GraphicDiffuseColor=[0.5 0.5 0.5]  GraphicSpecularColor=[0.5 0.5 0.5 1.0]  GraphicAmbientColor=[0.15 0.15 0.15 1.0]  GraphicEmissiveColor=[0.0 0.0 0.0 1.0]  GraphicShininess=75  GraphicOpacity=1.0
  InertiaOriginTransform : sm_lib/Frames and Transforms/Rigid Transform  TranslationMethod=Cartesian  TranslationStandardOffset=0  TranslationStandardOffsetUnits=m  TranslationStandardAxis=+Z  TranslationCartesianOffset=param_robot.link__2.d__inertiaOrigin  TranslationCartesianOffsetUnits=m  TranslationROffset=0  TranslationROffsetUnits=m  TranslationZOffset=0  TranslationZOffsetUnits=m  TranslationThetaOffset=0  TranslationThetaOffsetUnits=deg  RotationMethod=RotationMatrix  RotationAngleUnits=deg  RotationStandardAxis=+Z  RotationAngle=0.0  RotationArbitraryAxis=[0 0 1]  FollAlignAxisA=+X  BaseAlignAxisA=+Y  FollAlignAxisB=+Y  BaseAlignAxisB=+Z  RotationSequenceAxes=BaseAxes  RotationSequence=XYZ  RotationSequenceAngles=[0, 0, 0]  RotationSequenceAnglesUnits=rad  RotationMatrix=param_robot.link__2.R__inertiaOrigin  Quaternion=[1 0 0 0]
  ReferenceFrame : sm_lib/Frames and Transforms/Reference Frame
  Visual : sm_lib/Body Elements/File Solid  ExtGeomFileName=.\kukalbriiwa_model\meshes\link_2.stl  UnitType=Custom  ExtGeomFileUnits=mm  StepReaderType=HEX  ExportConvexHullGeometry=off  InertiaType=Custom  Mass=0  MassUnits=kg  CenterOfMass=[0, 0, 0]  CenterOfMassUnits=m  MomentsOfInertia=[0, 0, 0]  MomentsOfInertiaUnits=kg*m^2  ProductsOfInertia=[0, 0, 0]  ProductsOfInertiaUnits=kg*m^2  BasedOnType=Density  Density=1000  DensityUnits=kg/m^3  DoExposeReferenceFrame=on  SerializedFrames=<Frames/>  GraphicType=FromGeometry  MarkerShape=Sphere  MarkerSize=10  GraphicVisPropType=SimpleVisualProperties  GraphicDiffuseColor=[1, 0.423529411765, 0.0392156862745]  GraphicSpecularColor=[0.5 0.5 0.5 1.0]  GraphicAmbientColor=[0.15 0.15 0.15 1.0]  GraphicEmissiveColor=[0.0 0.0 0.0 1.0]  GraphicShininess=75  GraphicOpacity=1
  VisualOriginTransform : sm_lib/Frames and Transforms/Rigid Transform  TranslationMethod=Cartesian  TranslationStandardOffset=0  TranslationStandardOffsetUnits=m  TranslationStandardAxis=+Z  TranslationCartesianOffset=[0, 0, 0]  TranslationCartesianOffsetUnits=m  TranslationROffset=0  TranslationROffsetUnits=m  TranslationZOffset=0  TranslationZOffsetUnits=m  TranslationThetaOffset=0  TranslationThetaOffsetUnits=deg  RotationMethod=RotationSequence  RotationAngleUnits=deg  RotationStandardAxis=+Z  RotationAngle=0.0  RotationArbitraryAxis=[0 0 1]  FollAlignAxisA=+X  BaseAlignAxisA=+Y  FollAlignAxisB=+Y  BaseAlignAxisB=+Z  RotationSequenceAxes=BaseAxes  RotationSequence=XYZ  RotationSequenceAngles=[0, 0, 0]  RotationSequenceAnglesUnits=rad  RotationMatrix=[1 0 0; 0 1 0; 0 0 1]  Quaternion=[1 0 0 0]
  iiwa_joint_3_OriginTransform : sm_lib/Frames and Transforms/Rigid Transform  TranslationMethod=Cartesian  TranslationStandardOffset=0  TranslationStandardOffsetUnits=m  TranslationStandardAxis=+Z  TranslationCartesianOffset=param_robot.link__2.d__joint3  TranslationCartesianOffsetUnits=m  TranslationROffset=0  TranslationROffsetUnits=m  TranslationZOffset=0  TranslationZOffsetUnits=m  TranslationThetaOffset=0  TranslationThetaOffsetUnits=deg  RotationMethod=RotationMatrix  RotationAngleUnits=deg  RotationStandardAxis=+Z  RotationAngle=0.0  RotationArbitraryAxis=[0 0 1]  FollAlignAxisA=+X  BaseAlignAxisA=+Y  FollAlignAxisB=+Y  BaseAlignAxisB=+Z  RotationSequenceAxes=BaseAxes  RotationSequence=XYZ  RotationSequenceAngles=[1.57079632679, 0, -3.141592653589587]  RotationSequenceAnglesUnits=rad  RotationMatrix=param_robot.link__2.R__joint3  Quaternion=[1 0 0 0]
  F : PMIOPort  Side=Left
  F1 : PMIOPort  Port=2  Side=Right
  connections:
  iiwa_joint_3_OriginTransform/RConn1 -- F1/RConn1
  InertiaOriginTransform/LConn1 -- ReferenceFrame/RConn1 -- VisualOriginTransform/LConn1 -- F/RConn1 -- iiwa_joint_3_OriginTransform/LConn1
  Visual/RConn1 -- VisualOriginTransform/RConn1
  Inertia/RConn1 -- InertiaOriginTransform/RConn1

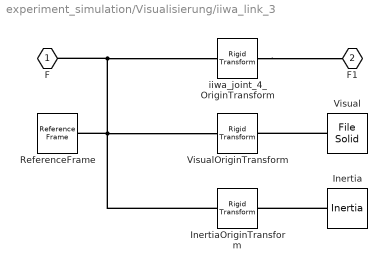
== system experiment_simulation/Visualisierung/iiwa_link_3 ==
  Inertia : sm_lib/Body Elements/Inertia  InertiaType=Custom  Mass=param_robot.link__3.m__3  MassUnits=kg  CenterOfMass=[0, 0, 0]  CenterOfMassUnits=m  MomentsOfInertia=param_robot.link__3.I__3  MomentsOfInertiaUnits=kg*m^2  ProductsOfInertia=[0, 0, 0]  ProductsOfInertiaUnits=kg*m^2  GraphicType=None  MarkerShape=Inertia  MarkerSize=20  GraphicVisPropType=SimpleVisualProperties  GraphicDiffuseColor=[0.5 0.5 0.5]  GraphicSpecularColor=[0.5 0.5 0.5 1.0]  GraphicAmbientColor=[0.15 0.15 0.15 1.0]  GraphicEmissiveColor=[0.0 0.0 0.0 1.0]  GraphicShininess=75  GraphicOpacity=1.0
  InertiaOriginTransform : sm_lib/Frames and Transforms/Rigid Transform  TranslationMethod=Cartesian  TranslationStandardOffset=0  TranslationStandardOffsetUnits=m  TranslationStandardAxis=+Z  TranslationCartesianOffset=param_robot.link__3.d__inertiaOrigin  TranslationCartesianOffsetUnits=m  TranslationROffset=0  TranslationROffsetUnits=m  TranslationZOffset=0  TranslationZOffsetUnits=m  TranslationThetaOffset=0  TranslationThetaOffsetUnits=deg  RotationMethod=RotationMatrix  RotationAngleUnits=deg  RotationStandardAxis=+Z  RotationAngle=0.0  RotationArbitraryAxis=[0 0 1]  FollAlignAxisA=+X  BaseAlignAxisA=+Y  FollAlignAxisB=+Y  BaseAlignAxisB=+Z  RotationSequenceAxes=BaseAxes  RotationSequence=XYZ  RotationSequenceAngles=[0, 0, 0]  RotationSequenceAnglesUnits=rad  RotationMatrix=param_robot.link__3.R__inertiaOrigin  Quaternion=[1 0 0 0]
  ReferenceFrame : sm_lib/Frames and Transforms/Reference Frame
  Visual : sm_lib/Body Elements/File Solid  ExtGeomFileName=.\kukalbriiwa_model\meshes\link_3.stl  UnitType=Custom  ExtGeomFileUnits=mm  StepReaderType=HEX  ExportConvexHullGeometry=off  InertiaType=Custom  Mass=0  MassUnits=kg  CenterOfMass=[0, 0, 0]  CenterOfMassUnits=m  MomentsOfInertia=[0, 0, 0]  MomentsOfInertiaUnits=kg*m^2  ProductsOfInertia=[0, 0, 0]  ProductsOfInertiaUnits=kg*m^2  BasedOnType=Density  Density=1000  DensityUnits=kg/m^3  DoExposeReferenceFrame=on  SerializedFrames=<Frames/>  GraphicType=FromGeometry  MarkerShape=Sphere  MarkerSize=10  GraphicVisPropType=SimpleVisualProperties  GraphicDiffuseColor=[1, 0.423529411765, 0.0392156862745]  GraphicSpecularColor=[0.5 0.5 0.5 1.0]  GraphicAmbientColor=[0.15 0.15 0.15 1.0]  GraphicEmissiveColor=[0.0 0.0 0.0 1.0]  GraphicShininess=75  GraphicOpacity=1
  VisualOriginTransform : sm_lib/Frames and Transforms/Rigid Transform  TranslationMethod=Cartesian  TranslationStandardOffset=0  TranslationStandardOffsetUnits=m  TranslationStandardAxis=+Z  TranslationCartesianOffset=[0, 0, 0]  TranslationCartesianOffsetUnits=m  TranslationROffset=0  TranslationROffsetUnits=m  TranslationZOffset=0  TranslationZOffsetUnits=m  TranslationThetaOffset=0  TranslationThetaOffsetUnits=deg  RotationMethod=RotationSequence  RotationAngleUnits=deg  RotationStandardAxis=+Z  RotationAngle=0.0  RotationArbitraryAxis=[0 0 1]  FollAlignAxisA=+X  BaseAlignAxisA=+Y  FollAlignAxisB=+Y  BaseAlignAxisB=+Z  RotationSequenceAxes=BaseAxes  RotationSequence=XYZ  RotationSequenceAngles=[0, 0, 0]  RotationSequenceAnglesUnits=rad  RotationMatrix=[1 0 0; 0 1 0; 0 0 1]  Quaternion=[1 0 0 0]
  iiwa_joint_4_OriginTransform : sm_lib/Frames and Transforms/Rigid Transform  TranslationMethod=Cartesian  TranslationStandardOffset=0  TranslationStandardOffsetUnits=m  TranslationStandardAxis=+Z  TranslationCartesianOffset=param_robot.link__3.d__joint4  TranslationCartesianOffsetUnits=m  TranslationROffset=0  TranslationROffsetUnits=m  TranslationZOffset=0  TranslationZOffsetUnits=m  TranslationThetaOffset=0  TranslationThetaOffsetUnits=deg  RotationMethod=RotationMatrix  RotationAngleUnits=deg  RotationStandardAxis=+Z  RotationAngle=0.0  RotationArbitraryAxis=[0 0 1]  FollAlignAxisA=+X  BaseAlignAxisA=+Y  FollAlignAxisB=+Y  BaseAlignAxisB=+Z  RotationSequenceAxes=BaseAxes  RotationSequence=XYZ  RotationSequenceAngles=[1.57079632679, 0, 0]  RotationSequenceAnglesUnits=rad  RotationMatrix=param_robot.link__3.R__joint4  Quaternion=[1 0 0 0]
  F : PMIOPort  Side=Left
  F1 : PMIOPort  Port=2  Side=Right
  connections:
  iiwa_joint_4_OriginTransform/RConn1 -- F1/RConn1
  InertiaOriginTransform/LConn1 -- ReferenceFrame/RConn1 -- VisualOriginTransform/LConn1 -- F/RConn1 -- iiwa_joint_4_OriginTransform/LConn1
  Visual/RConn1 -- VisualOriginTransform/RConn1
  Inertia/RConn1 -- InertiaOriginTransform/RConn1

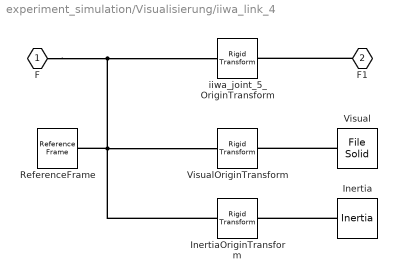
== system experiment_simulation/Visualisierung/iiwa_link_4 ==
  Inertia : sm_lib/Body Elements/Inertia  InertiaType=Custom  Mass=param_robot.link__4.m__4  MassUnits=kg  CenterOfMass=[0, 0, 0]  CenterOfMassUnits=m  MomentsOfInertia=param_robot.link__4.I__4  MomentsOfInertiaUnits=kg*m^2  ProductsOfInertia=[0, 0, 0]  ProductsOfInertiaUnits=kg*m^2  GraphicType=None  MarkerShape=Inertia  MarkerSize=20  GraphicVisPropType=SimpleVisualProperties  GraphicDiffuseColor=[0.5 0.5 0.5]  GraphicSpecularColor=[0.5 0.5 0.5 1.0]  GraphicAmbientColor=[0.15 0.15 0.15 1.0]  GraphicEmissiveColor=[0.0 0.0 0.0 1.0]  GraphicShininess=75  GraphicOpacity=1.0
  InertiaOriginTransform : sm_lib/Frames and Transforms/Rigid Transform  TranslationMethod=Cartesian  TranslationStandardOffset=0  TranslationStandardOffsetUnits=m  TranslationStandardAxis=+Z  TranslationCartesianOffset=param_robot.link__4.d__inertiaOrigin  TranslationCartesianOffsetUnits=m  TranslationROffset=0  TranslationROffsetUnits=m  TranslationZOffset=0  TranslationZOffsetUnits=m  TranslationThetaOffset=0  TranslationThetaOffsetUnits=deg  RotationMethod=RotationMatrix  RotationAngleUnits=deg  RotationStandardAxis=+Z  RotationAngle=0.0  RotationArbitraryAxis=[0 0 1]  FollAlignAxisA=+X  BaseAlignAxisA=+Y  FollAlignAxisB=+Y  BaseAlignAxisB=+Z  RotationSequenceAxes=BaseAxes  RotationSequence=XYZ  RotationSequenceAngles=[0, 0, 0]  RotationSequenceAnglesUnits=rad  RotationMatrix=param_robot.link__4.R__inertiaOrigin  Quaternion=[1 0 0 0]
  ReferenceFrame : sm_lib/Frames and Transforms/Reference Frame
  Visual : sm_lib/Body Elements/File Solid  ExtGeomFileName=.\kukalbriiwa_model\meshes\link_4.stl  UnitType=Custom  ExtGeomFileUnits=mm  StepReaderType=HEX  ExportConvexHullGeometry=off  InertiaType=Custom  Mass=0  MassUnits=kg  CenterOfMass=[0, 0, 0]  CenterOfMassUnits=m  MomentsOfInertia=[0, 0, 0]  MomentsOfInertiaUnits=kg*m^2  ProductsOfInertia=[0, 0, 0]  ProductsOfInertiaUnits=kg*m^2  BasedOnType=Density  Density=1000  DensityUnits=kg/m^3  DoExposeReferenceFrame=on  SerializedFrames=<Frames/>  GraphicType=FromGeometry  MarkerShape=Sphere  MarkerSize=10  GraphicVisPropType=SimpleVisualProperties  GraphicDiffuseColor=[1, 0.423529411765, 0.0392156862745]  GraphicSpecularColor=[0.5 0.5 0.5 1.0]  GraphicAmbientColor=[0.15 0.15 0.15 1.0]  GraphicEmissiveColor=[0.0 0.0 0.0 1.0]  GraphicShininess=75  GraphicOpacity=1
  VisualOriginTransform : sm_lib/Frames and Transforms/Rigid Transform  TranslationMethod=Cartesian  TranslationStandardOffset=0  TranslationStandardOffsetUnits=m  TranslationStandardAxis=+Z  TranslationCartesianOffset=[0, 0, 0]  TranslationCartesianOffsetUnits=m  TranslationROffset=0  TranslationROffsetUnits=m  TranslationZOffset=0  TranslationZOffsetUnits=m  TranslationThetaOffset=0  TranslationThetaOffsetUnits=deg  RotationMethod=RotationSequence  RotationAngleUnits=deg  RotationStandardAxis=+Z  RotationAngle=0.0  RotationArbitraryAxis=[0 0 1]  FollAlignAxisA=+X  BaseAlignAxisA=+Y  FollAlignAxisB=+Y  BaseAlignAxisB=+Z  RotationSequenceAxes=BaseAxes  RotationSequence=XYZ  RotationSequenceAngles=[0, 0, 0]  RotationSequenceAnglesUnits=rad  RotationMatrix=[1 0 0; 0 1 0; 0 0 1]  Quaternion=[1 0 0 0]
  iiwa_joint_5_OriginTransform : sm_lib/Frames and Transforms/Rigid Transform  TranslationMethod=Cartesian  TranslationStandardOffset=0  TranslationStandardOffsetUnits=m  TranslationStandardAxis=+Z  TranslationCartesianOffset=param_robot.link__4.d__joint5  TranslationCartesianOffsetUnits=m  TranslationROffset=0  TranslationROffsetUnits=m  TranslationZOffset=0  TranslationZOffsetUnits=m  TranslationThetaOffset=0  TranslationThetaOffsetUnits=deg  RotationMethod=RotationMatrix  RotationAngleUnits=deg  RotationStandardAxis=+Z  RotationAngle=0.0  RotationArbitraryAxis=[0 0 1]  FollAlignAxisA=+X  BaseAlignAxisA=+Y  FollAlignAxisB=+Y  BaseAlignAxisB=+Z  RotationSequenceAxes=BaseAxes  RotationSequence=XYZ  RotationSequenceAngles=[1.570796326799793, -2.068231071102144e-13, -3.141592653589793]  RotationSequenceAnglesUnits=rad  RotationMatrix=param_robot.link__4.R__joint5  Quaternion=[1 0 0 0]
  F : PMIOPort  Side=Left
  F1 : PMIOPort  Port=2  Side=Right
  connections:
  F1/RConn1 -- iiwa_joint_5_OriginTransform/RConn1
  Visual/RConn1 -- VisualOriginTransform/RConn1
  InertiaOriginTransform/LConn1 -- ReferenceFrame/RConn1 -- VisualOriginTransform/LConn1 -- F/RConn1 -- iiwa_joint_5_OriginTransform/LConn1
  Inertia/RConn1 -- InertiaOriginTransform/RConn1
